simulink model "simulation"  (R2019a)
settings: Solver=VariableStepAuto  StartTime=0.0  StopTime=10.0  RelTol=1e-3
values from neighbouring files (symbols this model uses):
  a = [0.328350063485 -0.504393436497 -18.7824329195 1.02511531984 -53.4041424252]    [a.mat]    (also in a1.mat = [-0.685212439995 -0.585400025674 -24.4194734415 0.9475851353; a2.mat = [-1.28043820376 -0.621828624231 -54.7528450797 1.71837449641; system_id.m = [A2(1) A1(1) A2(2) A1(2) A2(3)])
  b = [6.12465019513 -5.20663579301 6.03715613869 77.417940964 10.1407211952]    [b.mat]    (also in b1.mat = [34.2019090673 -33.7070179637 52.7248095782 336.319136551 44; b2.mat = [16.939936533 -14.6014953721 67.1462611587 436.465012222 564; system_id.m = [B2(1) B2(2) B1(1) B1(2) B2(3)])
undefined symbols (not defined in the file or in its folder): DiscIntNeverNeededParam
settings Model: Creator=ray  LastModifiedBy=ray
settings DebuggingCC: AlgebraicLoopMsg=none

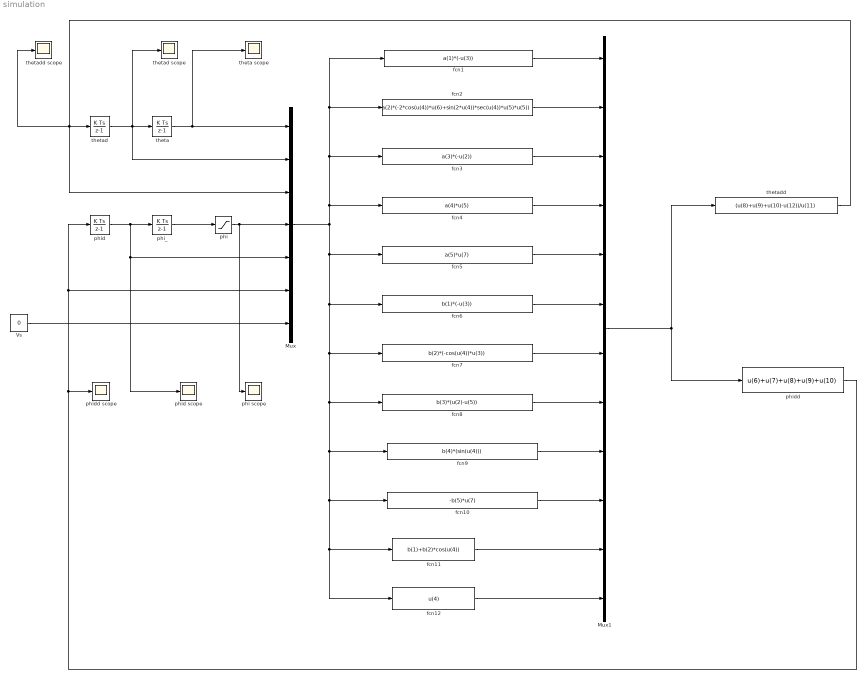
== system simulation ==
  Mux : Mux  Inputs=7
  Mux1 : Mux  Inputs=12
  Vs : Constant  Value=0
  fcn1 : Fcn  Expr=a(1)*(-u(3))
  fcn10 : Fcn  Expr=-b(5)*u(7)
  "fcn11 " : Fcn  Expr=b(1)+b(2)*cos(u(4))
  fcn12 : Fcn  Expr=u(4)
  fcn2 : Fcn  Expr=a(2)*(-2*cos(u(4))*u(6)+sin(2*u(4))*sec(u(4))*u(5)*u(5))
  fcn3 : Fcn  Expr=a(3)*(-u(2))
  fcn4 : Fcn  Expr=a(4)*u(5)
  fcn5 : Fcn  Expr=a(5)*u(7)
  fcn6 : Fcn  Expr=b(1)*(-u(3))
  fcn7 : Fcn  Expr=b(2)*(-cos(u(4))*u(3))
  fcn8 : Fcn  Expr=b(3)*(u(2)-u(5))
  fcn9 : Fcn  Expr=b(4)*(sin(u(4)))
  phi : Saturate  UpperLimit=1.6  LowerLimit=-1.6
  "phi scope " : Scope
  phi_ : DiscreteIntegrator  InitialCondition=pi/180  SampleTime=0.001  ICPrevOutput=DiscIntNeverNeededParam  ICPrevScaledInput=DiscIntNeverNeededParam
  phid : DiscreteIntegrator  SampleTime=0.001  ICPrevOutput=DiscIntNeverNeededParam  ICPrevScaledInput=DiscIntNeverNeededParam
  "phid scope " : Scope
  phidd : Fcn  Expr=u(6)+u(7)+u(8)+u(9)+u(10)
  "phidd scope " : Scope
  theta : DiscreteIntegrator  SampleTime=0.001  ICPrevOutput=DiscIntNeverNeededParam  ICPrevScaledInput=DiscIntNeverNeededParam
  theta scope : Scope
  thetad : DiscreteIntegrator  SampleTime=0.001  ICPrevOutput=DiscIntNeverNeededParam  ICPrevScaledInput=DiscIntNeverNeededParam
  "thetad scope " : Scope
  thetadd : Fcn  Expr=(u(8)+u(9)+u(10)-u(12))/u(11)
  "thetadd scope " : Scope
  wires:
  phid/1 -> "phid scope "/1, Mux/5, phi_/1
  phi_/1 -> phi/1
  phi/1 -> Mux/4, "phi scope "/1
  phidd/1 -> "phidd scope "/1, Mux/6, phid/1
  Vs/1 -> Mux/7
  fcn8/1 -> Mux1/8
  fcn7/1 -> Mux1/7
  fcn6/1 -> Mux1/6
  fcn5/1 -> Mux1/5
  fcn4/1 -> Mux1/4
  fcn3/1 -> Mux1/3
  fcn2/1 -> Mux1/2
  fcn1/1 -> Mux1/1
  fcn9/1 -> Mux1/9
  theta/1 -> theta scope/1, Mux/1
  Mux1/1 -> thetadd/1, phidd/1
  fcn10/1 -> Mux1/10
  "fcn11 "/1 -> Mux1/11
  fcn12/1 -> Mux1/12
  Mux/1 -> fcn1/1, fcn2/1, fcn3/1, fcn4/1, fcn12/1, "fcn11 "/1, fcn10/1, fcn9/1, fcn8/1, fcn7/1, fcn6/1, fcn5/1
  thetad/1 -> "thetad scope "/1, Mux/2, theta/1
  thetadd/1 -> "thetadd scope "/1, Mux/3, thetad/1
